simulink subsystem "PvtSubSys_LSM"  (R2020b)
settings: Solver=VariableStepAuto  StartTime=0.0  StopTime=10.0  RelTol=1e-3
values from neighbouring files (symbols this model uses):
  P_LSM_ALC_Enable = 0.0    [LSM_Parameter.sldd]
  P_LSM_DOP_C0_EN_Limit = 0.8    [LSM_Parameter.sldd]
  P_LSM_DOP_C0_out_Limit = 2.0    [LSM_Parameter.sldd]
  P_LSM_DOP_C1_EN_Limit : value not decoded    [LSM_Parameter.sldd]
  P_LSM_DOP_C1_out_Limit : value not decoded    [LSM_Parameter.sldd]
  P_LSM_DOP_C1AndC2_Lim_X : value not decoded    [LSM_Parameter.sldd]
  P_LSM_DOP_C2_EN_Limit : value not decoded    [LSM_Parameter.sldd]
  P_LSM_DOP_C2_out_Limit : value not decoded    [LSM_Parameter.sldd]
  P_LSM_DOP_In_Pre2Dop_Dis = 1.0    [LSM_Parameter.sldd]
  P_LSM_DOP_Out_Pre2Dop_Dis = 2.0    [LSM_Parameter.sldd]
  P_LSM_DOP_PreDis_X : value not decoded    [LSM_Parameter.sldd]
  P_LSM_DOP_PreDis_Y : value not decoded    [LSM_Parameter.sldd]
  P_LSM_DOPValid_CheckTime = 0.06    [LSM_Parameter.sldd]
  P_LSM_DoubleLine_Curr2Cent_Dislimit = 0.5    [LSM_Parameter.sldd]
  P_LSM_DoubleLine_Dop2Cent_Dislimit = 0.5    [LSM_Parameter.sldd]
  P_LSM_DoubleLine_DOPOut_C1 : value not decoded    [LSM_Parameter.sldd]
  P_LSM_DoubleLine_Pre2Cent_Dislimit = 1.0    [LSM_Parameter.sldd]
  P_LSM_IFV2CenterAxis = 0.0    [LSM_Parameter.sldd]
  P_LSM_IFV2RearAxis = 0.0    [LSM_Parameter.sldd]
  P_LSM_LineSTD_Limit = 0.15    [LSM_Parameter.sldd]
  P_LSM_NOH_Switch = 0.0    [LSM_Parameter.sldd]
  P_LSM_Pre_t = 0.0    [LSM_Parameter.sldd]
  P_LSM_SingleLine_Cent2Edge_Dislimit = 100.0    [LSM_Parameter.sldd]
  P_LSM_SingleLine_Curr2Cent_Dislimit = 0.2    [LSM_Parameter.sldd]
  P_LSM_SingleLine_Dop2Cent_Dislimit = 0.2    [LSM_Parameter.sldd]
  P_LSM_SingleLine_DOPOut_C1 : value not decoded    [LSM_Parameter.sldd]
  P_LSM_SingleLine_Pre2Cent_Dislimit = 0.5    [LSM_Parameter.sldd]
undefined symbols (not defined in the file or in its folder): P_LSM_LineWijCal_C12, P_LSM_LineWijCal_C13, P_LSM_PosLineLcFac
libraries: simulink x92, TrueDurationTime x2
(part 3 of 9)

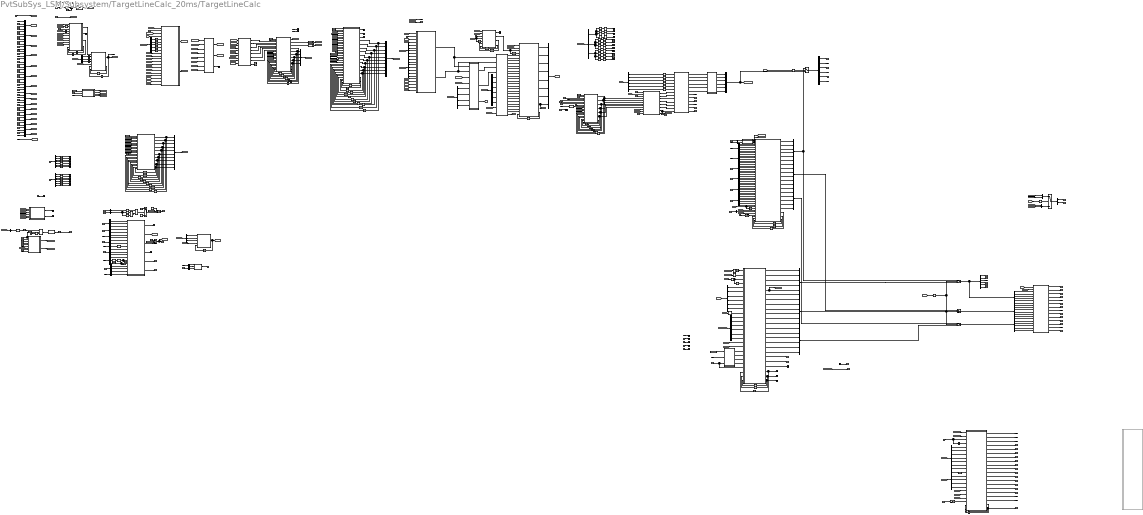
== system PvtSubSys_LSM/Subsystem/TargetLineCalc_20ms/TargetLineCalc ==
  kap : Inport
  vRef : Inport  Port=2
  OTLineValid : Inport  Port=3
  aOTL : Inport  Port=4
  bOTL : Inport  Port=5
  cOTL : Inport  Port=6
  dOTL : Inport  Port=7
  dxMax : Inport  Port=8
  OTLCount : Inport  Port=9
  ACCMode : Inport  Port=10
  HWASts : Inport  Port=11
  LRELineUpdate : Inport  Port=12
  LALineUpdate : Inport  Port=13
  LeftLine_Change : Inport  Port=14
  RightLine_Change : Inport  Port=15
  L1_Conf : Inport  Port=16
  L2_Conf : Inport  Port=17
  L3_Conf : Inport  Port=18
  L4_Conf : Inport  Port=19
  L1_A3 : Inport  Port=20
  L2_A3 : Inport  Port=21
  L3_A3 : Inport  Port=22
  L4_A3 : Inport  Port=23
  L1_A2 : Inport  Port=24
  L2_A2 : Inport  Port=25
  L3_A2 : Inport  Port=26
  L4_A2 : Inport  Port=27
  L1_A1 : Inport  Port=28
  L2_A1 : Inport  Port=29
  L3_A1 : Inport  Port=30
  L4_A1 : Inport  Port=31
  L1_A0 : Inport  Port=32
  L2_A0 : Inport  Port=33
  L3_A0 : Inport  Port=34
  L4_A0 : Inport  Port=35
  L1_R : Inport  Port=36
  L2_R : Inport  Port=37
  L3_R : Inport  Port=38
  L4_R : Inport  Port=39
  L1_Re : Inport  Port=40
  L2_Re : Inport  Port=41
  L3_Re : Inport  Port=42
  L4_Re : Inport  Port=43
  Edge1_R : Inport  Port=44
  Edge2_R : Inport  Port=45
  Edge1_A3 : Inport  Port=46
  Edge2_A3 : Inport  Port=47
  Edge1_A2 : Inport  Port=48
  Edge2_A2 : Inport  Port=49
  Edge1_A1 : Inport  Port=50
  Edge2_A1 : Inport  Port=51
  Edge1_A0 : Inport  Port=52
  Edge2_A0 : Inport  Port=53
  Edge1_Conf : Inport  Port=54
  Edge2_Conf : Inport  Port=55
  Edge1_Re : Inport  Port=56
  Edge2_Re : Inport  Port=57
  LeftLineType : Inport  Port=58
  RightLineType : Inport  Port=59
  LeftDLM : Inport  Port=60
  RightDLM : Inport  Port=61
  LH1Color : Inport  Port=62
  LH2Color : Inport  Port=63
  LeftDECELType : Inport  Port=64
  RightDECELType : Inport  Port=65
  LLeftType : Inport  Port=66
  pathPredValid : Inport  Port=67
  pathPredC3 : Inport  Port=68
  pathPredC2 : Inport  Port=69
  pathPredC1 : Inport  Port=70
  pathPredC0 : Inport  Port=71
  ESSSts : Inport  Port=72
  LCKSts : Inport  Port=73
  RFM_INTERSEC_ALERT : Inport  Port=74
  RFM_CURRENT_LANE : Inport  Port=75
  RFM_RIGHT_LANE : Inport  Port=76
  RFM_BRANCH : Inport  Port=77
  RFM_ROAD : Inport  Port=78  OutDataTypeStr=Bus: RFM_ROAD_BUS  PortDimensions=1  BusOutputAsStruct=on
  RFM_LINE_ENTRY_CL : Inport  Port=79
  RFM_LINE_EXIT_CL : Inport  Port=80
  RFM_LINE_CL : Inport  Port=81
  RFM_TSR_BUS : Inport  Port=82  OutDataTypeStr=Bus: RFM_TSR_BUS
  RFM_REC_LANES : Inport  Port=83
  RFM_LINE_L1 : Inport  Port=84
  RFM_LINE_R1 : Inport  Port=85
  RFM_LINE_L2 : Inport  Port=86
  RFM_LINE_R2 : Inport  Port=87
  Bus Creator : BusCreator  Inputs=10
  Bus Creator1 : BusCreator  Inputs=10
  Bus Creator10 : BusCreator  Inputs=2
  Bus Creator11 : BusCreator  Inputs=5
  Bus Creator12 : BusCreator  Inputs=8
  Bus Creator{2..8} (7 alike) : BusCreator  Inputs=6
  Bus Creator9 : BusCreator  Inputs=2
  Bus Selector : BusSelector  OutputSignals=LineConf,A1,A0
  Bus Selector1 : BusSelector  OutputSignals=LineConf
  Bus Selector{2,9..10,39} (4 alike) : BusSelector  OutputSignals=HWALineValid,HWALineC3,HWALineC2,HWALineC1,HWALineC0,HWARange
  Bus Selector11 : BusSelector  OutputSignals=b_is_avalible,en_lane_type
  Bus Selector12 : BusSelector  OutputSignals=b_is_available,f_distance,en_direction
  Bus Selector13 : BusSelector  OutputSignals=i_mapvalid
  Bus Selector14 : BusSelector  OutputSignals=nLaneNum,nLaneID
  Bus Selector15 : BusSelector  OutputSignals=b_vanish_valid
  Bus Selector{7,16,20..21,29} (5 alike) : BusSelector  OutputSignals=bIsLineExist,dC0V,dC1V,dC2V,dC3V,dDisFront
  Bus Selector17 : BusSelector  OutputSignals=dDisStart,bIsLineExist,dC0V
  Bus Selector18 : BusSelector  OutputSignals=bIsLineExist,dC0V,dC1V,dC2V,dC3V,dDisStart,dDisFront
  Bus Selector19 : BusSelector  OutputSignals=bIsLineExist,dC0V,dC1V,dC2V,dC3V,dDisStart,dDisFront
  Bus Selector22 : BusSelector  OutputSignals=Avail_time,Avail_dis,A0
  Bus Selector23 : BusSelector  OutputSignals=PathValid,PathA3,PathA2,PathA1,PathA0,PathRange
  Bus Selector24 : BusSelector  OutputSignals=RoadType
  Bus Selector25 : BusSelector  OutputSignals=HWALeLineValid,HWALeLineC3,HWALeLineC2,HWALeLineC1,HWALeLineC0,HWALeRange
  Bus Selector26 : BusSelector  OutputSignals=i_rec_lanes_num,i_rec_lanes
  Bus Selector27 : BusSelector  OutputSignals=eLineType
  Bus Selector28 : BusSelector  OutputSignals=eLineType
  Bus Selector3 : BusSelector  OutputSignals=LineConf,A3,A2,A1,A0,Range,tLost
  Bus Selector30 : BusSelector  OutputSignals=LineConf,A3,A2,A1,A0,LineReliable,Range
  Bus Selector31 : BusSelector  OutputSignals=RoadType,VehInLeftmostLane,VehInRightmostLane
  Bus Selector32 : BusSelector  OutputSignals=i_mapvalid,i_on_nav_path
  Bus Selector33 : BusSelector  OutputSignals=bIsLineExist,dDisStart,dC0V
  Bus Selector34 : BusSelector  OutputSignals=SPL_LaneChanged
  Bus Selector35 : BusSelector  OutputSignals=f_vanish_pt_dis
  Bus Selector36 : BusSelector  OutputSignals=HWARiLineValid,HWARiLineC3,HWARiLineC2,HWARiLineC1,HWARiLineC0,HWARiRange
  Bus Selector37 : BusSelector  OutputSignals=b_is_avalible
  Bus Selector38 : BusSelector  OutputSignals=LineValid,A3,A2,A1,A0
  Bus Selector4 : BusSelector  OutputSignals=EdgeConf,EdgeA3,EdgeA2,EdgeA1,EdgeA0
  Bus Selector40 : BusSelector  OutputSignals=LeftEn,RightEn
  Bus Selector41 : BusSelector  OutputSignals=LineValid,A3,A2,A1,A0
  Bus Selector42 : BusSelector  OutputSignals=LineConf,A3,A2,A1,A0,Range
  Bus Selector43 : BusSelector  OutputSignals=A3,A2,A1,A0
  Bus Selector5 : BusSelector  OutputSignals=EdgeConf,EdgeA1,EdgeA0
  Bus Selector6 : BusSelector  OutputSignals=PathValid,PathA3,PathA2,PathA1,PathA0,PathRange
  Bus Selector8 : BusSelector  OutputSignals=bIsLineExist,dC0V,dC1V,dC2V,dC3V,dDisFront,dDisStart
  CalcEgoVehMove : MATLAB Function  TreatAsAtomicUnit=on
  CalcEgoVehMove2 : MATLAB Function  TreatAsAtomicUnit=on
  Compare To Constant10 : simulink/Logic and Bit Operations/Compare To Constant  relop===  const=2  OutDataTypeStr=boolean
  Compare To Constant17 : simulink/Logic and Bit Operations/Compare To Constant  relop=~=  const=0  OutDataTypeStr=boolean
  Compare To Constant2 : simulink/Logic and Bit Operations/Compare To Constant  relop=~=  const=0  OutDataTypeStr=boolean
  Compare To Constant3 : simulink/Logic and Bit Operations/Compare To Constant  relop=~=  const=0  OutDataTypeStr=boolean
  Compare To Constant8 : simulink/Logic and Bit Operations/Compare To Constant  relop=>  const=0  OutDataTypeStr=boolean
  Compare To Constant9 : simulink/Logic and Bit Operations/Compare To Constant  relop===  const=1  OutDataTypeStr=boolean
  Compare To Zero : simulink/Logic and Bit Operations/Compare To Zero  relop=>  OutDataTypeStr=boolean
  Compare To Constant1 : simulink/Logic and Bit Operations/Compare To Constant  relop===  const=0  OutDataTypeStr=boolean
  Compare To Constant59 : simulink/Logic and Bit Operations/Compare To Constant  relop=~=  const=2  OutDataTypeStr=boolean
  Compare To Constant60 : simulink/Logic and Bit Operations/Compare To Constant  relop=>=  const=150  OutDataTypeStr=boolean
  Constant{,1..4} (5 alike) : Constant  Value=0.02  OutDataTypeStr=single
  Constant10 : Constant  Value=P_LSM_NOH_Switch
  Constant14 : Constant  Value=P_LSM_LineSTD_Limit
  Constant15 : Constant  Value=0  OutDataTypeStr=uint8
  Constant16 : Constant  Value=3  OutDataTypeStr=uint8
  Constant17 : Constant  Value=0  OutDataTypeStr=uint8
  Constant18 : Constant  Value=P_LSM_ALC_Enable  OutDataTypeStr=uint8
  Constant7 : Constant  Value=P_LSM_Pre_t
  Constant8 : Constant  Value=1.3  OutDataTypeStr=single
  Constant9 : Constant  Value=2  OutDataTypeStr=uint8
  D1 : Lookup_n-D  NumberOfTableDimensions=1  BreakpointsForDimension1=[0,30,40]  Table=[10,25,25]  InternalRulePriority=Speed  RndMeth=Simplest  InputSameDT=on
  D2 : Lookup_n-D  NumberOfTableDimensions=1  BreakpointsForDimension1=[0,30,40]  Table=[15,25,25]  InternalRulePriority=Speed  RndMeth=Simplest  InputSameDT=on
  Data Type Conversion{,1..3} (4 alike) : DataTypeConversion  OutDataTypeStr=boolean
  DetectChange : Subsystem
  DetectIncrease : Subsystem
  DetectIncrease1 : Subsystem
  ESSLineCalc : MATLAB Function  Commented=on  TreatAsAtomicUnit=on
  ESSLineCalc1 : MATLAB Function  TreatAsAtomicUnit=on
  Gain3 : Gain  Gain=3.6
  Gain4 : Gain  Gain=1.03
  Ground : Ground
  HWALineCalc : MATLAB Function  TreatAsAtomicUnit=on
  LCKSts1 : InportShadow  Port=73
  LH1Color1 : InportShadow  Port=62
  LREWidthCalc : MATLAB Function  TreatAsAtomicUnit=on
  LeftLineType1 : InportShadow  Port=58
  LineSelect : MATLAB Function  TreatAsAtomicUnit=on
  Logical Operator : Logic  Inputs=3  AllPortsSameDT=off  OutDataTypeStr=boolean
  Logical Operator7 : Logic  AllPortsSameDT=off  OutDataTypeStr=boolean
  Logical Operator8 : Logic  Operator=OR  AllPortsSameDT=off  OutDataTypeStr=boolean
  MATLAB Function : MATLAB Function  TreatAsAtomicUnit=on
  MATLAB Function1 : MATLAB Function  TreatAsAtomicUnit=on
  MATLAB Function2 : MATLAB Function  TreatAsAtomicUnit=on
  MATLAB Function3 : MATLAB Function  TreatAsAtomicUnit=on
  MATLAB Function4 : MATLAB Function  TreatAsAtomicUnit=on
  MATLAB Function5 : MATLAB Function  TreatAsAtomicUnit=on
  MATLAB Function6 : MATLAB Function  TreatAsAtomicUnit=on
  Mux{,1..6} (7 alike) : Mux
  Mux{7..15} (9 alike) : Mux  Inputs=2
  NOA : MATLAB Function  TreatAsAtomicUnit=on
  RFM_CURRENT_LANE1 : InportShadow  Port=75
  RFM_CURRENT_LANE2 : InportShadow  Port=75
  RFM_LINE_ENTRY_CL1 : InportShadow  Port=79
  RFM_LINE_EXIT_CL1 : InportShadow  Port=80
  RFM_LINE_EXIT_CL2 : InportShadow  Port=80
  RFM_LINE_L3 : InportShadow  Port=84
  RFM_LINE_R3 : InportShadow  Port=85
  RFM_ROAD1 : InportShadow  Port=78  OutDataTypeStr=Bus: RFM_ROAD_BUS  PortDimensions=1  BusOutputAsStruct=on
  RFM_ROAD2 : InportShadow  Port=78  OutDataTypeStr=Bus: RFM_ROAD_BUS  PortDimensions=1  BusOutputAsStruct=on
  RFM_TSR_BUS1 : InportShadow  Port=82  OutDataTypeStr=Bus: RFM_TSR_BUS
  RFM_TSR_BUS2 : InportShadow  Port=82  OutDataTypeStr=Bus: RFM_TSR_BUS
  RightLineType1 : InportShadow  Port=59
  RoadWidthCalc1 : MATLAB Function  TreatAsAtomicUnit=on
  Selector : Selector  InputPortWidth=4  IndexOptions=Index vector (dialog)  Indices=2  OutputSizes=1
  Selector{1,4..5,10} (4 alike) : Selector  InputPortWidth=4  IndexOptions=Index vector (dialog)  Indices=1  OutputSizes=1
  Selector11 : Selector  InputPortWidth=4  IndexOptions=Index vector (dialog)  Indices=4  OutputSizes=1
  Selector12 : Selector  InputPortWidth=4  IndexOptions=Index vector (dialog)  Indices=3  OutputSizes=1
  Selector{13..18} (6 alike) : Selector  InputPortWidth=3  IndexOptions=Index vector (dialog)  Indices=2  OutputSizes=1
  Selector2 : Selector  InputPortWidth=4  IndexOptions=Index vector (dialog)  Indices=3  OutputSizes=1
  Selector3 : Selector  InputPortWidth=4  IndexOptions=Index vector (dialog)  Indices=2  OutputSizes=1
  Selector6 : Selector  InputPortWidth=4  IndexOptions=Index vector (dialog)  Indices=4  OutputSizes=1
  Selector7 : Selector  InputPortWidth=4  IndexOptions=Index vector (dialog)  Indices=4  OutputSizes=1
  Selector8 : Selector  InputPortWidth=4  IndexOptions=Index vector (dialog)  Indices=3  OutputSizes=1
  Selector9 : Selector  InputPortWidth=4  IndexOptions=Index vector (dialog)  Indices=2  OutputSizes=1
  Signal Copy{,1..3,8,10..35} (31 alike) : SignalConversion  OverrideOpt=off
  Subsystem2 : Subsystem
  Subsystem3 : Subsystem
  Subsystem4 : Subsystem
  Subsystem5 : Subsystem
  Sum : Sum  Inputs=|++
  Switch{,1..6,9} (8 alike) : Switch  Criteria=u2 > Threshold
  TJA2NOA : MATLAB Function  TreatAsAtomicUnit=on
  Terminator{,1..49} (50 alike) : Terminator
  TrueDurationTime : TrueDurationTime/TrueDurationTime  TCycle=0.02
  TypeConf : Subsystem
  TypeConf1 : Subsystem
  Unit Delay{,1,6,10,13,15,27,30..32,34..35,39..41,49..52,58..59,64} (22 alike) : UnitDelay  SampleTime=-1  HasFrameUpgradeWarning=on
  Unit Delay11 : UnitDelay  InitialCondition=uint8(0)  SampleTime=-1  HasFrameUpgradeWarning=on
  Unit Delay12 : UnitDelay  InitialCondition=int8(0)  SampleTime=-1  HasFrameUpgradeWarning=on
  Unit Delay14 : UnitDelay  InitialCondition=3.75  SampleTime=-1  HasFrameUpgradeWarning=on
  Unit Delay16 : UnitDelay  InitialCondition=uint8(0)  SampleTime=-1  HasFrameUpgradeWarning=on
  Unit Delay{17..22,38} (7 alike) : UnitDelay  InitialCondition=single(zeros(2,1))  SampleTime=-1  HasFrameUpgradeWarning=on
  Unit Delay2 : UnitDelay  InitialCondition=[5;5;5;5]  SampleTime=-1  HasFrameUpgradeWarning=on
  Unit Delay23 : UnitDelay  InitialCondition=uint8(zeros(2,1))  SampleTime=-1  HasFrameUpgradeWarning=on
  Unit Delay24 : UnitDelay  InitialCondition=uint8(0)  SampleTime=-1  HasFrameUpgradeWarning=on
  Unit Delay25 : UnitDelay  InitialCondition=false  SampleTime=-1  HasFrameUpgradeWarning=on
  Unit Delay26 : UnitDelay  InitialCondition=int8(0)  SampleTime=-1  HasFrameUpgradeWarning=on
  Unit Delay{4..5,7..9,28..29,37,57,60..61} (11 alike) : UnitDelay  InitialCondition=zeros(4,1)  SampleTime=-1  HasFrameUpgradeWarning=on
  Unit Delay33 : UnitDelay  InitialCondition=3.75  SampleTime=-1  HasFrameUpgradeWarning=on
  Unit Delay36 : UnitDelay  InitialCondition=8  SampleTime=-1  HasFrameUpgradeWarning=on
  Unit Delay42 : UnitDelay  InitialCondition=false  SampleTime=-1  HasFrameUpgradeWarning=on
  Unit Delay{43..48,54,56,66..70} (13 alike) : UnitDelay  InitialCondition=single(0)  SampleTime=-1  HasFrameUpgradeWarning=on
  Unit Delay55 : UnitDelay  InitialCondition=false  SampleTime=-1  HasFrameUpgradeWarning=on
  Unit Delay62 : UnitDelay  InitialCondition=zeros(2,1)  SampleTime=-1  HasFrameUpgradeWarning=on
  Unit Delay63 : UnitDelay  InitialCondition=zeros(2,1)  SampleTime=-1  HasFrameUpgradeWarning=on
  Unit Delay65 : UnitDelay  InitialCondition=int8(0)  SampleTime=-1  HasFrameUpgradeWarning=on
  VehStation : MATLAB Function  TreatAsAtomicUnit=on
  VisLineFilter1 : MATLAB Function  TreatAsAtomicUnit=on
  VisLineFilter2 : MATLAB Function  TreatAsAtomicUnit=on
  VisLineFilter3 : MATLAB Function  TreatAsAtomicUnit=on
  VisLineFilter4 : MATLAB Function  TreatAsAtomicUnit=on
  VisLineFilter5 : MATLAB Function  TreatAsAtomicUnit=on
  YBranchRi : MATLAB Function  TreatAsAtomicUnit=on
  kap1 : InportShadow
  kap2 : InportShadow
  kap4 : InportShadow
  preDisMinTable : Lookup_n-D  NumberOfTableDimensions=1  BreakpointsForDimension1=[0 5 10 15 20 25 30 35 40 60 80 90 100 110 120 140]  Table=[8 9 10 11 12 13 14 15 17 22 28 31 35 38 42 49]  ExtrapMethod=Clip  InternalRulePriority=Speed  RndMeth=Simplest  InputSameDT=on
  tFilt : Constant  Value=0.2  OutDataTypeStr=single
  vRef{1..12,14} (13 alike) : InportShadow  Port=2
  TJALineValid : Outport
  TJALineA3 : Outport  Port=2
  TJALineA2 : Outport  Port=3
  TJALineA1 : Outport  Port=4
  TJALineA0 : Outport  Port=5
  TJALineRange : Outport  Port=6
  LCKLineValid : Outport  Port=7
  LCKLineA3 : Outport  Port=8
  LCKLineA2 : Outport  Port=9
  LCKLineA1 : Outport  Port=10
  LCKLineA0 : Outport  Port=11
  LCKLineRange : Outport  Port=12
  HWALineValid : Outport  Port=13
  HWALineA3 : Outport  Port=14
  HWALineA2 : Outport  Port=15
  HWALineA1 : Outport  Port=16
  HWALineA0 : Outport  Port=17
  HWALineRange : Outport  Port=18
  HWALineLValid1 : Outport  Port=19
  HWALineLA3 : Outport  Port=20
  HWALineLA2 : Outport  Port=21
  HWALineLA1 : Outport  Port=22
  HWALineLA0 : Outport  Port=23
  HWALineLRange : Outport  Port=24
  HWALineRValid : Outport  Port=25
  HWALineRA3 : Outport  Port=26
  HWALineRA2 : Outport  Port=27
  HWALineRA1 : Outport  Port=28
  HWALineRA0 : Outport  Port=29
  HWALineRRange0 : Outport  Port=30
  pre_dy_Error : Outport  Port=31
  pre_HeadAng_Error : Outport  Port=32
  MLeLane : Outport  Port=33
  RoadWidth : Outport  Port=34
  SingleLineLost_b : Outport  Port=35
  DoubleLineLost_b : Outport  Port=36
  LeLineCrossing : Outport  Port=37
  RiLineCrossing : Outport  Port=38
  MRiLane : Outport  Port=39
  MrcStopLane : Outport  Port=40
  HWALeLineVirtual : Outport  Port=41
  HWARiLineVirtual : Outport  Port=42
  LeLineLcAvailable : Outport  Port=43
  RiLineLcAvailable : Outport  Port=44
  ESSLineValid : Outport  Port=45
  ESSLineA3 : Outport  Port=46
  ESSLineA2 : Outport  Port=47
  ESSLineA1 : Outport  Port=48
  ESSLineA0 : Outport  Port=49
  ESSLineRange : Outport  Port=50
  ESSLineLValid : Outport  Port=51
  ESSLineLA3 : Outport  Port=52
  ESSLineLA2 : Outport  Port=53
  ESSLineLA1 : Outport  Port=54
  ESSLineLA0 : Outport  Port=55
  ESSLineLRange : Outport  Port=56
  ESSLineRValid : Outport  Port=57
  ESSLineRA3 : Outport  Port=58
  ESSLineRA2 : Outport  Port=59
  ESSLineRA1 : Outport  Port=60
  ESSLineRA0 : Outport  Port=61
  ESSLineRRange : Outport  Port=62
  ESSLineLock_b : Outport  Port=63
  leftLaneCurise_b : Outport  Port=64
  PilotSts : Outport  Port=65
  PilotTurnSwSts : Outport  Port=66
  PilotSPLDist : Outport  Port=67
  PilotSPL : Outport  Port=68
  TJALineSource : Outport  Port=69
  tag scope: RoadWidth=global, VisEdge=global, VisLine=global
  wires:
  [LH2Wij] -> VisLineFilter2/21(LH2Wij)
  [LH1Wij] -> VisLineFilter2/20(LH1Wij)
  Unit Delay35/1 -> RoadWidthCalc1/4(a0)
  Unit Delay59/1 -> RoadWidthCalc1/3(a1)
  Unit Delay58/1 -> RoadWidthCalc1/2(VisLineConf)
  Bus Selector/2 -> Unit Delay59/1  "<A1>"
  Bus Selector/1 -> Unit Delay58/1  "<LineConf>"
  Unit Delay13/1 -> YBranchRi/2(RightOffset_b)
  YBranchRi/2(YBranchRi_b) -> Terminator48/1
  Unit Delay12/1 -> VisLineFilter5/28(LockIDK1)
  VisLineFilter5/9(LockID) -> Unit Delay12/1
  MATLAB Function3/8(Line_State) -> Terminator41/1
  [RightOffset_b] -> VisLineFilter2/19(RightLineChange)
  [LeftOffset_b] -> VisLineFilter2/18(LeftLineChange)
  Ground/1 -> SingleLineLost_b/1  "SingleLineLost_b"
  kap1/1 -> Subsystem2/12(kap)
  Bus Selector37/1 -> MATLAB Function/3(Right_avail)  "<b_is_avalible>"
  RFM_RIGHT_LANE/1 -> Bus Selector37/1
  Bus Selector11/2 -> MATLAB Function/2(Cur_LaneType)  "<en_lane_type>"
  RFM_CURRENT_LANE2/1 -> Bus Selector11/1
  MATLAB Function/1(MrcStopLane) -> MrcStopLane/1
  Bus Selector11/1 -> MATLAB Function/1(Cur_avail)  "<b_is_avalible>"
  Subsystem2/7(TJA_Line_State) -> [TJA_Line_State], LineSelect/13(TJA_Line_State)  "LSM_TJA_Line_State"
  Subsystem2/6(OTL_Range) -> LineSelect/12(dxMax)
  Subsystem2/2(OTL_C3) -> LineSelect/8(aOTL)
  Subsystem2/1(OTL_Valid) -> LineSelect/7(OTLineValid)
  Subsystem2/4(OTL_C1) -> LineSelect/10(cOTL)
  Subsystem2/5(OTL_C0) -> LineSelect/11(dOTL)
  Subsystem2/3(OTL_C2) -> LineSelect/9(bOTL)
  [VisEdge] -> Subsystem2/11(EdgeLine)
  [CentLine] -> Subsystem2/10(CentLine)
  vRef2/1 -> Subsystem2/3(vRef)  "LSM_VRef"
  LCKSts1/1 -> Subsystem2/1(LCKSts)
  VisLineFilter1/3(A2) -> Unit Delay48/1, Subsystem2/6(DOP_C2)
  VisLineFilter1/5(A0) -> Subsystem2/8(DOP_C0), Unit Delay46/1
  VisLineFilter1/4(A1) -> Subsystem2/7(DOP_C1), Unit Delay47/1
  Unit Delay46/1 -> VisLineFilter1/18(A0K1)
  VisLineFilter1/7(tLost) -> Unit Delay44/1
  VisLineFilter1/6(Range) -> Subsystem2/9(DOP_Range), Unit Delay45/1
  Unit Delay44/1 -> VisLineFilter1/20(tLostK1)
  Unit Delay47/1 -> VisLineFilter1/17(A1K1)
  Unit Delay42/1 -> VisLineFilter1/14(LineValidK1)
  Unit Delay48/1 -> VisLineFilter1/16(A2K1)
  VisLineFilter1/1(LineValid) -> Subsystem2/4(DOP_Valid), Unit Delay42/1
  Unit Delay43/1 -> VisLineFilter1/15(A3K1)
  Unit Delay45/1 -> VisLineFilter1/19(RangeK1)
  VisLineFilter1/2(A3) -> Subsystem2/5(DOP_C3), Unit Delay43/1
  Constant2/1 -> VisLineFilter1/1(tCycle)
  aOTL/1 -> VisLineFilter1/4(aOTL)
  bOTL/1 -> VisLineFilter1/5(bOTL)
  cOTL/1 -> VisLineFilter1/6(cOTL)
  dxMax/1 -> VisLineFilter1/8(R)
  [dDeltaX] -> VisLineFilter1/10(dDeltaX)
  [dDeltaY] -> VisLineFilter1/11(dDeltaY)
  [CosOfPsi] -> VisLineFilter1/12(CosOfPsi)
  [SinOfPsi] -> VisLineFilter1/13(SinOfPsi)
  Unit Delay23/1 -> VisLineFilter4/15(EdgeConfK1)
  Unit Delay22/1 -> VisLineFilter4/17(EdgeA3K1)
  Unit Delay21/1 -> VisLineFilter4/18(EdgeA2K1)
  VisLineFilter4/1(EdgeConf) -> Unit Delay23/1, Bus Creator/1
  VisLineFilter4/3(EdgeA3) -> Unit Delay22/1, Bus Creator/3
  VisLineFilter4/4(EdgeA2) -> Bus Creator/4, Unit Delay21/1
  Unit Delay20/1 -> VisLineFilter4/19(EdgeA1K1)
  VisLineFilter4/5(EdgeA1) -> Bus Creator/5, Unit Delay20/1
  Unit Delay19/1 -> VisLineFilter4/20(EdgeA0K1)
  VisLineFilter4/6(EdgeA0) -> Bus Creator/6, Unit Delay19/1
  Unit Delay18/1 -> VisLineFilter4/21(EdgeRangeK1)
  VisLineFilter4/7(EdgeRange) -> Bus Creator/7, Unit Delay18/1
  Unit Delay17/1 -> VisLineFilter4/22(EdgetLostK1)
  [VisEdgeConf] -> VisLineFilter4/2(VisEdgeConf)
  Constant4/1 -> VisLineFilter4/1(tCycle)
  [VisEdgeA3] -> VisLineFilter4/4(a3)
  [VisEdgeA2] -> VisLineFilter4/5(a2)
  [VisEdgeA1] -> VisLineFilter4/6(a1)
  [VisEdgeA0] -> VisLineFilter4/7(a0)
  [VisEdgeRange] -> VisLineFilter4/8(R)
  [VisEdgeUpdate] -> VisLineFilter4/9(LineUpdate)
  [dDeltaX] -> VisLineFilter4/10(dDeltaX)
  [dDeltaY] -> VisLineFilter4/11(dDeltaY)
  [CosOfPsi] -> VisLineFilter4/12(CosOfPsi)
  [SinOfPsi] -> VisLineFilter4/13(SinOfPsi)
  vRef6/1 -> VisLineFilter4/14(vRef)  "LSM_VRef"
  LALineUpdate/1 -> [VisLineUpdate]
  LRELineUpdate/1 -> [VisEdgeUpdate]
  OTLineValid/1 -> VisLineFilter1/3(OTLineValid)
  OTLCount/1 -> DetectChange/1(OTLCount)
  DetectChange/1(Out1) -> VisLineFilter1/9(LineUpdate)
  Bus Creator/1 -> [VisEdge]
  ESSSts/1 -> ESSLineCalc1/3(ESSSts), Unit Delay24/1
  [VisLine] -> Bus Selector3/1
  Bus Selector3/3 -> ESSLineCalc1/7(A2)  "<A2>"
  Bus Selector3/2 -> ESSLineCalc1/6(A3)  "<A3>"
  Bus Selector3/1 -> ESSLineCalc1/5(LineConf)  "<LineConf>"
  [VisEdge] -> Bus Selector4/1
  Bus Selector4/2 -> ESSLineCalc1/13(EdgeA3)  "<EdgeA3>"
  Bus Selector4/1 -> Data Type Conversion1/1  "<EdgeConf>"
  Bus Selector4/3 -> ESSLineCalc1/14(EdgeA2)  "<EdgeA2>"
  [LeftOffset_b] -> ESSLineCalc1/17(LeftOffset_b)
  [RightOffset_b] -> ESSLineCalc1/18(RightOffset_b)
  [RoadWidth] -> ESSLineCalc1/19(RoadWidth)
  vRef3/1 -> D1/1  "LSM_VRef"
  D1/1 -> ESSLineCalc1/20(ESSDistLim)
  ESSLineCalc1/20(Lock_b) -> ESSLineLock_b/1, Unit Delay25/1
  Unit Delay25/1 -> ESSLineCalc1/22(Lock_bK1)
  ESSLineCalc1/19(MoveID) -> Unit Delay26/1
  Unit Delay26/1 -> ESSLineCalc1/21(MoveIDK1)
  ESSLineCalc1/17(ESSRiLineA0) -> ESSLineRA0/1
  ESSLineCalc1/16(ESSRiLineA1) -> ESSLineRA1/1
  ESSLineCalc1/15(ESSRiLineA2) -> ESSLineRA2/1
  ESSLineCalc1/14(ESSRiLineA3) -> ESSLineRA3/1
  ESSLineCalc1/11(ESSLeLineA0) -> ESSLineLA0/1
  ESSLineCalc1/1(ESSLineValid) -> ESSLineValid/1
  ESSLineCalc1/6(ESSRange) -> ESSLineRange/1
  ESSLineCalc1/7(ESSLeLineValid) -> ESSLineLValid/1
  ESSLineCalc1/2(ESSLineA3) -> ESSLineA3/1
  ESSLineCalc1/3(ESSLineA2) -> ESSLineA2/1
  ESSLineCalc1/4(ESSLineA1) -> ESSLineA1/1
  ESSLineCalc1/5(ESSLineA0) -> ESSLineA0/1
  ESSLineCalc1/8(ESSLeLineA3) -> ESSLineLA3/1
  ESSLineCalc1/9(ESSLeLineA2) -> ESSLineLA2/1
  ESSLineCalc1/10(ESSLeLineA1) -> ESSLineLA1/1
  ESSLineCalc1/12(ESSLeRange) -> ESSLineLRange/1
  ESSLineCalc1/13(ESSRiLineValid) -> ESSLineRValid/1
  ESSLineCalc1/18(ESSRiRange) -> ESSLineRRange/1
  Data Type Conversion1/1 -> ESSLineCalc1/12(EdgeValid)
  Unit Delay24/1 -> ESSLineCalc1/4(ESSStsK1)
  vRef/1 -> VisLineFilter2/15(vRef)  "LSM_VRef"
  [VisLineA3] -> VisLineFilter2/5(a3)
  VisLineFilter2/8(A1) -> Bus Creator1/5, Unit Delay7/1
  VisLineFilter2/6(A3) -> Bus Creator1/3, Unit Delay9/1
  VisLineFilter2/7(A2) -> Bus Creator1/4, Unit Delay8/1
  [CosOfPsi] -> VisLineFilter2/13(CosOfPsi)
  VisLineFilter2/11(tLost) -> Bus Creator1/8, Unit Delay2/1
  [SinOfPsi] -> VisLineFilter2/14(SinOfPsi)
  VisLineFilter2/3(DevDis) -> Terminator6/1
  [VisLineUpdate] -> VisLineFilter2/10(LineUpdate)
  Constant3/1 -> VisLineFilter2/2(tCycle)
  VisLineFilter2/2(DevAngle) -> Terminator5/1
  [VisLineA1] -> VisLineFilter2/7(a1)
  tFilt/1 -> VisLineFilter2/1(tF)
  VisLineFilter2/10(Range) -> Bus Creator1/7, Unit Delay4/1
  Unit Delay57/1 -> VisLineFilter2/22(LineConfK1)
  [dDeltaX] -> VisLineFilter2/11(dDeltaX)
  Unit Delay8/1 -> VisLineFilter2/25(A2K1)
  Unit Delay9/1 -> VisLineFilter2/24(A3K1)
  Unit Delay7/1 -> VisLineFilter2/26(A1K1)
  [VisLineR] -> VisLineFilter2/9(R)
  [VisLineConf] -> VisLineFilter2/3(VisLineConf)
  VisLineFilter2/1(DevValid) -> Terminator4/1
  Unit Delay5/1 -> VisLineFilter2/27(A0K1)
  VisLineFilter2/9(A0) -> Bus Creator1/6, Unit Delay5/1
  Bus Creator1/1 -> [VisLine]
  [VisLineA0] -> VisLineFilter2/8(a0)
  [RoadWidth] -> VisLineFilter2/17(RoadWidth)
  [dDeltaY] -> VisLineFilter2/12(dDeltaY)
  VisLineFilter2/4(LineConf) -> Bus Creator1/1, Unit Delay57/1
  Unit Delay2/1 -> VisLineFilter2/29(tLostK1)
  Unit Delay4/1 -> VisLineFilter2/28(RangeK1)
  [VisLineA2] -> VisLineFilter2/6(a2)
  YBranchRi/1(YBranch_b) -> RoadWidthCalc1/1(YBranch_b)
  [VisLineConf] -> YBranchRi/9(Conf)
  HWALineCalc/18(HWARiRange) -> Bus Creator7/6
  [VisLine] -> Bus Selector1/1
  Unit Delay34/1 -> YBranchRi/12(DistRiK1)
  Compare To Constant1/1 -> Logical Operator/1
  YBranchRi/4(DistRi) -> Unit Delay34/1
  Compare To Constant60/1 -> leftLaneCurise_b/1  "leftLaneCurise_b"
  Logical Operator/1 -> TrueDurationTime/1
  Compare To Constant59/1 -> Logical Operator/2
  [VisLineA2] -> YBranchRi/6(A2)
  TypeConf/1(Out1) -> [LeftLineTypeEN]  "LSM_LeftLineTypeEN"
  HWALineCalc/17(HWARiLineC0) -> Bus Creator7/5
  [RoadWidth] -> Unit Delay33/1
  HWALineCalc/19(preDyDiff) -> pre_dy_Error/1
  YBranchRi/3(Dist) -> Unit Delay32/1
  vRef12/1 -> YBranchRi/3(vRef)  "LSM_VRef"
  HWALineCalc/15(HWARiLineC2) -> Bus Creator7/3
  HWALineCalc/21(Error) -> Terminator/1
  RoadWidthCalc1/2(tLost) -> Unit Delay15/1
  RoadWidthCalc1/1(RoadWidth) -> RoadWidth/1, [RoadWidth], Unit Delay14/1
  [VisLineUpdate] -> RoadWidthCalc1/5(LineUpdate)
  [VisLineA1] -> YBranchRi/7(A1)
  [RightOffset_b] -> HWALineCalc/19(RightOffset_b)
  RightLineType/1 -> TypeConf/4(RightType)
  Unit Delay30/1 -> HWALineCalc/25(MoveIDK1)
  [LeftOffset_b] -> HWALineCalc/18(LeftOffset_b)
  HWALineCalc/16(HWARiLineC1) -> Bus Creator7/4
  CalcEgoVehMove2/2(dDeltaY) -> HWALineCalc/21(dDeltaY)
  Compare To Zero/1 -> Logical Operator/3
  Selector1/1 -> Compare To Constant1/1
  vRef7/1 -> HWALineCalc/24(vRef), CalcEgoVehMove2/3(Vego)  "LSM_VRef"
  HWALineCalc/20(HeadAngDiff) -> pre_HeadAng_Error/1
  Unit Delay16/1 -> HWALineCalc/4(HWAStsK1)
  vRef5/1 -> Compare To Zero/1  "LSM_VRef"
  Unit Delay15/1 -> RoadWidthCalc1/7(tLostK1)
  CalcEgoVehMove2/3(CosOfPsi) -> HWALineCalc/22(CosOfPsi)
  TrueDurationTime/1 -> Compare To Constant60/1
  Unit Delay33/1 -> YBranchRi/4(RoadWidth)
  Constant7/1 -> CalcEgoVehMove2/1(tCycle)
  [VisLineA3] -> YBranchRi/5(A3)
  kap4/1 -> CalcEgoVehMove2/2(Kap)
  CalcEgoVehMove2/4(SinOfPsi) -> HWALineCalc/23(SinOfPsi)
  [HWASts] -> Signal Copy/1
  Unit Delay14/1 -> RoadWidthCalc1/6(RoadWidthK1)
  HWALineCalc/14(HWARiLineC3) -> Bus Creator7/2
  TypeConf/2(Out2) -> [RightLineTypeEN]  "LSM_RightLineTypeEN"
  Bus Selector1/1 -> Selector1/1  "<LineConf>"
  [RightOffset_b] -> Unit Delay13/1
  HWALineCalc/13(HWARiLineValid) -> Bus Creator7/1
  [VisLine] -> Bus Selector/1
  LeftLineType/1 -> TypeConf/1(LeftType), Compare To Constant59/1
  [VisLineUpdate] -> YBranchRi/1(LineUpdate)
  HWALineCalc/22(MoveID) -> Terminator28/1, Unit Delay30/1  "LSM_MoveID"
  Unit Delay32/1 -> YBranchRi/11(DistK1)
  [VisLineA0] -> YBranchRi/8(A0)
  CalcEgoVehMove2/1(dDeltaX) -> HWALineCalc/20(dDeltaX)
  Constant/1 -> CalcEgoVehMove/1(tCycle)
  CalcEgoVehMove/1(dDeltaX) -> [dDeltaX]
  CalcEgoVehMove/3(CosOfPsi) -> [CosOfPsi]
  CalcEgoVehMove/4(SinOfPsi) -> [SinOfPsi]
  CalcEgoVehMove/2(dDeltaY) -> [dDeltaY]
  vRef1/1 -> CalcEgoVehMove/3(Vego)  "LSM_VRef"
  kap/1 -> CalcEgoVehMove/2(Kap)
  LeftDLM/1 -> TypeConf/2(LeftDLMType)
  RightDLM/1 -> TypeConf/5(RightDLMType)
  Bus Selector5/1 -> LREWidthCalc/1(LRELineConf)  "<EdgeConf>"
  Unit Delay36/1 -> LREWidthCalc/5(LREWidthK1)
  [VisEdge] -> Bus Selector5/1
  [VisEdgeUpdate] -> LREWidthCalc/4(LRELineUpdate)
  LREWidthCalc/1(LREWidth) -> [LREWidth], Unit Delay36/1
  [VisLineReliable] -> VisLineFilter2/4(VisLineReliable)
  VisLineFilter2/5(LineReliable) -> Bus Creator1/2, Unit Delay37/1
  Unit Delay37/1 -> VisLineFilter2/23(LineReliableK1)
  [VisEdgeReliable] -> VisLineFilter4/3(VisEdgeReliable)
  VisLineFilter4/2(EdgeReliable) -> Unit Delay38/1, Bus Creator/2
  Unit Delay38/1 -> VisLineFilter4/16(EdgeReliableK1)
  VisLineFilter4/8(EdgetLost) -> Unit Delay17/1, Bus Creator/8
  Bus Selector/3 -> Unit Delay35/1  "<A0>"
  Bus Selector5/2 -> LREWidthCalc/2(a1)  "<EdgeA1>"
  Bus Selector5/3 -> LREWidthCalc/3(a0)  "<EdgeA0>"
  Bus Selector3/4 -> ESSLineCalc1/8(A1)  "<A1>"
  Bus Selector3/5 -> ESSLineCalc1/9(A0)  "<A0>"
  Bus Selector3/6 -> ESSLineCalc1/10(Range)  "<Range>"
  Bus Selector3/7 -> ESSLineCalc1/11(tLost)  "<tLost>"
  Bus Selector4/4 -> ESSLineCalc1/15(EdgeA1)  "<EdgeA1>"
  Bus Selector4/5 -> ESSLineCalc1/16(EdgeA0)  "<EdgeA0>"
  Compare To Constant2/1 -> Switch3/2, Switch2/2, Switch/2
  HWALineCalc/3(HWALineC2) -> Bus Creator4/3
  HWALineCalc/6(HWARange) -> Bus Creator4/6
  Bus Creator3/1 -> Switch2/3
  Bus Selector10/1 -> HWALineValid/1  "<HWALineValid>"
  HWALineCalc/2(HWALineC3) -> Bus Creator4/2
  Bus Creator4/1 -> Switch/3
  HWALineCalc/9(HWALeLineC2) -> Bus Creator3/3
  Bus Selector10/2 -> HWALineA3/1  "<HWALineC3>"
  Bus Selector9/2 -> TJALineA3/1  "<HWALineC3>"
  HWALineCalc/12(HWALeRange) -> Bus Creator3/6
  HWALineCalc/5(HWALineC0) -> [HWALineC0], Bus Creator4/5
  Bus Selector10/6 -> HWALineRange/1  "<HWARange>"
  HWALineCalc/1(HWALineValid) -> Bus Creator4/1
  Bus Selector9/1 -> TJALineValid/1  "<HWALineValid>"
  Bus Selector10/3 -> HWALineA2/1  "<HWALineC2>"
  Bus Selector9/4 -> TJALineA1/1  "<HWALineC1>"
  Bus Selector9/3 -> TJALineA2/1  "<HWALineC2>"
  Bus Selector9/5 -> TJALineA0/1  "<HWALineC0>"
  Bus Creator2/1 -> Switch1/3, [TJA_Line]
  Switch1/1 -> Bus Selector9/1
  Bus Selector9/6 -> TJALineRange/1  "<HWARange>"
  HWALineCalc/8(HWALeLineC3) -> Bus Creator3/2
  HWALineCalc/10(HWALeLineC1) -> Bus Creator3/4
  HWALineCalc/11(HWALeLineC0) -> Bus Creator3/5
  HWALineCalc/7(HWALeLineValid) -> Bus Creator3/1
  Bus Selector10/5 -> HWALineA0/1  "<HWALineC0>"
  HWALineCalc/4(HWALineC1) -> Bus Creator4/4
  Bus Selector10/4 -> HWALineA1/1  "<HWALineC1>"
  TJA2NOA/1(HWALineValid) -> Bus Creator2/1
  TJA2NOA/2(HWALineC3) -> Bus Creator2/2
  TJA2NOA/3(HWALineC2) -> Bus Creator2/3
  TJA2NOA/4(HWALineC1) -> Bus Creator2/4
  TJA2NOA/5(HWALineC0) -> Bus Creator2/5
  TJA2NOA/6(HWARange) -> Bus Creator2/6
  VisLineFilter2/13(Avail_dis) -> Bus Creator1/10, Unit Delay60/1
  Unit Delay60/1 -> VisLineFilter2/31(Avail_disK1)
  VisLineFilter2/12(Avail_time) -> Bus Creator1/9, Unit Delay61/1
  Unit Delay61/1 -> VisLineFilter2/30(Avail_timeK1)
  Constant14/1 -> VisLineFilter2/16(Lowlimit)
  RFM_INTERSEC_ALERT/1 -> Bus Selector12/1
  RFM_ROAD/1 -> Bus Selector13/1
  Bus Selector12/1 -> Subsystem3/1(Intersec_available)  "<b_is_available>"
  Bus Selector12/2 -> Subsystem3/2(f_distance)  "<f_distance>"
  Bus Selector12/3 -> Subsystem3/3(en_direction)  "<en_direction>"
  Subsystem3/1(PilotRoadSts) -> Terminator42/1  "LSM_PilotTurnSwSts"
  Subsystem3/2(PilotTurnSwSts) -> [PilotRoadSts]  "LSM_PilotRoadSts"
  Subsystem3/3(PilotSts) -> Switch4/3  "LSM_PilotSts"
  [VisEdgeA0] -> VehStation/5(VisEdgeA0)
  [VisLineA0] -> VehStation/2(VisLineA0)
  [VisEdgeConf] -> VehStation/4(VisEdgeConf)
  [VisLineType] -> VehStation/3(VisLineType)
  [VisLineConf] -> VehStation/1(VisLineConf)
  Signal Copy8/1 -> Subsystem3/15(VehInLeftmostLane), MLeLane/1  "LSM_LeftMostLane"
  [PilotSts] -> Compare To Constant3/1
  RFM_LINE_ENTRY_CL/1 -> Bus Selector18/1
  RFM_LINE_EXIT_CL/1 -> Bus Selector17/1
  Subsystem3/6(PilotSPLDist) -> PilotSPLDist/1  "LSM_PilotSPLDist"
  Subsystem3/5(LSM_PilotSPL) -> PilotSPL/1  "LSM_PilotSPL"
  Bus Selector18/1 -> Signal Copy10/1  "<bIsLineExist>"
  Signal Copy10/1 -> Terminator1/1  "LSM_EN_Valid"
  Bus Selector18/4 -> Signal Copy13/1  "<dC2V>"
  Bus Selector18/3 -> Signal Copy12/1  "<dC1V>"
  Bus Selector18/2 -> Signal Copy11/1  "<dC0V>"
  Bus Selector18/5 -> Signal Copy14/1  "<dC3V>"
  Bus Selector18/6 -> Signal Copy15/1  "<dDisStart>"
  Bus Selector18/7 -> Signal Copy16/1  "<dDisFront>"
  Signal Copy11/1 -> Terminator7/1  "LSM_EN_C0"
  Signal Copy12/1 -> Terminator8/1  "LSM_EN_C1"
  Signal Copy13/1 -> Terminator9/1  "LSM_EN_C2"
  Signal Copy14/1 -> Terminator10/1  "LSM_EN_C3"
  Signal Copy15/1 -> Terminator11/1  "LSM_EN_Start"
  Signal Copy16/1 -> Terminator12/1  "LSM_EN_Front"
  Signal Copy23/1 -> Terminator16/1  "LSM_Exit_Front"
  Signal Copy22/1 -> Terminator15/1  "LSM_Exit_Start"
  Signal Copy21/1 -> Terminator14/1  "LSM_Exit_C3"
  Signal Copy20/1 -> Terminator19/1  "LSM_Exit_C2"
  Signal Copy19/1 -> Terminator18/1  "LSM_Exit_C1"
  Signal Copy18/1 -> Terminator17/1  "LSM_Exit_C0"
  Bus Selector19/7 -> Signal Copy23/1  "<dDisFront>"
  Bus Selector19/6 -> Signal Copy22/1  "<dDisStart>"
  Bus Selector19/5 -> Signal Copy21/1  "<dC3V>"
  Bus Selector19/2 -> Signal Copy18/1  "<dC0V>"
  Bus Selector19/3 -> Signal Copy19/1  "<dC1V>"
  Bus Selector19/4 -> Signal Copy20/1  "<dC2V>"
  Signal Copy17/1 -> Terminator13/1  "LSM_Exit_Valid"
  Bus Selector19/1 -> Signal Copy17/1  "<bIsLineExist>"
  RFM_LINE_EXIT_CL1/1 -> Bus Selector19/1
  VisLineFilter4/9(Avail_time) -> Bus Creator/9, Unit Delay63/1
  VisLineFilter4/10(Avail_dis) -> Bus Creator/10, Unit Delay62/1
  Unit Delay62/1 -> VisLineFilter4/24(Avail_disK1)
  Unit Delay63/1 -> VisLineFilter4/23(Avail_timeK1)
  HWALineCalc/24(Lock_counter) -> Terminator30/1, Unit Delay64/1  "LSM_LockCounter"
  Unit Delay64/1 -> HWALineCalc/27(Lock_counterK1)
  Unit Delay65/1 -> HWALineCalc/26(LockIDK1)
  HWALineCalc/23(LockID) -> Terminator29/1, Unit Delay65/1  "LSM_LockID"
  [VisLine] -> Bus Selector22/1
  Selector/1 -> Signal Copy25/1
  Selector2/1 -> Signal Copy24/1
  Bus Selector22/2 -> Selector4/1, Selector3/1, Selector7/1, Selector8/1  "<Avail_dis>"
  Selector4/1 -> Signal Copy26/1
  Selector3/1 -> Signal Copy27/1
  Signal Copy25/1 -> Terminator20/1  "LSM_L2_AvaliTime"
  Signal Copy24/1 -> Terminator21/1  "LSM_L3_AvaliTime"
  Signal Copy26/1 -> Terminator22/1  "LSM_L1_AvaliDis"
  Signal Copy27/1 -> Terminator23/1  "LSM_L2_AvaliDis"
  Signal Copy28/1 -> Terminator24/1  "LSM_L1_AvaliTime"
  Selector5/1 -> Signal Copy28/1
  Bus Selector22/1 -> Selector5/1, Selector/1, Selector2/1, Selector6/1  "<Avail_time>"
  Signal Copy29/1 -> Terminator25/1  "LSM_L4_AvaliTime"
  Selector6/1 -> Signal Copy29/1
  Signal Copy31/1 -> Terminator27/1  "LSM_L4_AvaliDis"
  Signal Copy30/1 -> Terminator26/1  "LSM_L3_AvaliDis"
  Selector7/1 -> Signal Copy31/1
  Selector8/1 -> Signal Copy30/1
  Selector12/1 -> Signal Copy34/1
  Selector11/1 -> Signal Copy35/1
  Signal Copy34/1 -> Terminator33/1  "LSM_L3_A0"
  Signal Copy35/1 -> Terminator34/1  "LSM_L4_A0"
  Signal Copy33/1 -> Terminator32/1  "LSM_L2_A0"
  Signal Copy32/1 -> Terminator31/1  "LSM_L1_A0"
  Selector9/1 -> Signal Copy33/1
  Selector10/1 -> Signal Copy32/1
  Bus Selector22/3 -> Selector12/1, Selector11/1, Selector9/1, Selector10/1  "<A0>"
  [LeftLineTypeEN] -> ESSLineCalc1/1(LeftLineTypeEn)
  [RightLineTypeEN] -> ESSLineCalc1/2(RightLineTypeEn)
  Unit Delay27/1 -> HWALineCalc/1(HWALineC0K1)  "LSM_HWALineC0K1"
  [VisLineReliable] -> YBranchRi/10(Reliable)
  VisLineFilter2/15(Fault) -> Unit Delay29/1
  VisLineFilter2/14(fix_time) -> Unit Delay28/1
  Unit Delay28/1 -> VisLineFilter2/32(fix_timeK1)
  Unit Delay29/1 -> VisLineFilter2/33(FaultK1)
  vRef11/1 -> Gain3/1  "LSM_VRef"
  Constant8/1 -> Sum/2
  Gain4/1 -> Sum/1
  Gain3/1 -> Gain4/1
  Sum/1 -> preDisMinTable/1
  preDisMinTable/1 -> [preDis]
  dOTL/1 -> VisLineFilter1/7(dOTL)
  vRef14/1 -> VisLineFilter1/2(vRef)  "LSM_VRef"
  [Line_State] -> Subsystem2/2(Line_State)
  kap2/1 -> [kap]
  LCKSts/1 -> MATLAB Function6/3(LCKSts)
  Switch4/1 -> [PilotSts], PilotSts/1
  Constant9/1 -> Switch4/1
  Constant10/1 -> Switch4/2
  [VisLineColor] -> VehStation/6(VisLineColor)
  VisLineFilter3/1(DoubleLineLost_b) -> [Double_Line_Lost]
  [Double_Line_Lost] -> DoubleLineLost_b/1  "DoubleLineLost_b"
  pathPredValid/1 -> Terminator36/1
  pathPredC3/1 -> Terminator37/1
  pathPredC2/1 -> Terminator38/1
  pathPredC1/1 -> Terminator39/1
  pathPredC0/1 -> Terminator40/1
  [CentLine] -> Bus Selector23/1
  Bus Selector23/3 -> HWALineCalc/7(PathA2)  "<PathA2>"
  Bus Selector23/2 -> HWALineCalc/6(PathA3)  "<PathA3>"
  Bus Selector23/4 -> HWALineCalc/8(PathA1)  "<PathA1>"
  Bus Selector23/1 -> HWALineCalc/5(PathValid)  "<PathValid>"
  Bus Selector23/5 -> HWALineCalc/9(PathA0)  "<PathA0>"
  Bus Selector23/6 -> HWALineCalc/10(PathRange)  "<PathRange>"
  Compare To Constant8/1 -> Logical Operator7/1
  Bus Selector24/1 -> Compare To Constant10/1, Compare To Constant9/1  "<RoadType>"
  Compare To Constant9/1 -> Logical Operator8/1
  Compare To Constant10/1 -> Logical Operator8/2
  Logical Operator7/1 -> Switch5/2
  Constant15/1 -> Switch5/1
  Switch5/1 -> Switch6/3
  Logical Operator8/1 -> Logical Operator7/2
  Constant16/1 -> Switch5/3
  Bus Selector13/1 -> Compare To Constant8/1  "<i_mapvalid>"
  RFM_TSR_BUS/1 -> Bus Selector24/1
  Switch6/1 -> PilotTurnSwSts/1
  Constant17/1 -> Switch6/1
  Constant18/1 -> Switch6/2
  RFM_REC_LANES/1 -> Bus Selector26/1
  Bus Selector26/1 -> Subsystem3/4(i_rec_lanes_num)  "<i_rec_lanes_num>"
  Bus Selector26/2 -> Subsystem3/5(i_rec_lanes)  "<i_rec_lanes>"
  RFM_ROAD1/1 -> Bus Selector14/1
  Bus Selector14/1 -> Subsystem3/6(nLaneNum)  "<nLaneNum>"
  Bus Selector14/2 -> Subsystem3/7(nLaneID)  "<nLaneID>"
  RFM_CURRENT_LANE/1 -> Bus Selector15/1
  Bus Selector15/1 -> Data Type Conversion/1  "<b_vanish_valid>"
  RFM_BRANCH/1 -> Terminator43/1
  Subsystem3/4(LaneChange) -> Terminator44/1
  Bus Selector8/7 -> NOA/33(Exit_Start)  "<dDisStart>"
  Bus Selector16/5 -> NOA/38(RFM_LineCL_A3)  "<dC3V>"
  Bus Selector21/6 -> NOA/26(RFM_LineR2_Range)  "<dDisFront>"
  Bus Selector7/3 -> NOA/11(RFM_LineL2_A1)  "<dC1V>"
  Bus Selector28/1 -> TypeConf1/2(RightType)  "<eLineType>"
  Unit Delay41/1 -> NOA/48(Lock_counterK1)
  RFM_LINE_CL/1 -> Bus Selector16/1
  RFM_LINE_R3/1 -> Bus Selector20/1
  NOA/21(Lock_counter) -> Unit Delay41/1
  Bus Selector20/1 -> NOA/15(RFM_LineR1_Valid)  "<bIsLineExist>"
  RFM_LINE_R1/1 -> Bus Selector28/1
  Bus Selector8/5 -> NOA/31(Exit_A3)  "<dC3V>"
  Bus Selector34/1 -> NOA/43(LaneChange)  "<SPL_LaneChanged>"
  NOA/4(HWALineC1) -> Bus Creator5/4
  RFM_LINE_L1/1 -> Bus Selector27/1
  NOA/5(HWALineC0) -> Bus Creator5/5
  Bus Selector20/4 -> NOA/18(RFM_LineR1_A2)  "<dC2V>"
  Bus Selector27/1 -> TypeConf1/1(LeftType)  "<eLineType>"
  RFM_LINE_L3/1 -> Bus Selector29/1
  Bus Selector8/1 -> NOA/27(Exit_Valid)  "<bIsLineExist>"
  Bus Selector8/4 -> NOA/30(Exit_A2)  "<dC2V>"
  NOA/17(HWARiLineC0) -> Bus Creator8/5
  Bus Selector16/2 -> NOA/35(RFM_LineCL_A0)  "<dC0V>"
  TypeConf1/2(RightEn) -> [RFM_RiLineLcAvailable], NOA/2(RightEn)
  Bus Selector21/5 -> NOA/25(RFM_LineR2_A3)  "<dC3V>"
  RFM_LINE_R2/1 -> Bus Selector21/1
  Bus Selector8/3 -> NOA/29(Exit_A1)  "<dC1V>"
  Bus Selector16/4 -> NOA/37(RFM_LineCL_A2)  "<dC2V>"
  Bus Selector8/2 -> NOA/28(Exit_A0)  "<dC0V>"
  NOA/15(HWARiLineC2) -> Bus Creator8/3
  Bus Selector20/6 -> NOA/20(RFM_LineR1_Range)  "<dDisFront>"
  Bus Selector7/6 -> NOA/14(RFM_LineL2_Range)  "<dDisFront>"
  Bus Selector21/4 -> NOA/24(RFM_LineR2_A2)  "<dC2V>"
  Bus Selector21/1 -> NOA/21(RFM_LineR2_Valid)  "<bIsLineExist>"
  Bus Selector8/6 -> NOA/32(Exit_Range)  "<dDisFront>"
  Bus Selector20/3 -> NOA/17(RFM_LineR1_A1)  "<dC1V>"
  RFM_LINE_EXIT_CL2/1 -> Bus Selector8/1
  Bus Selector16/1 -> NOA/34(RFM_LineCL_Valid)  "<bIsLineExist>"
  Bus Selector29/2 -> NOA/4(RFM_LineL1_A0)  "<dC0V>"
  RFM_LINE_L2/1 -> Bus Selector7/1
  [HWASts] -> Unit Delay39/1, NOA/40(HWASts)
  NOA/7(HWALeLineValid) -> Bus Creator6/1
  Bus Selector29/1 -> NOA/3(RFM_LineL1_Valid)  "<bIsLineExist>"
  Bus Selector21/3 -> NOA/23(RFM_LineR2_A1)  "<dC1V>"
  Unit Delay39/1 -> NOA/41(HWAStsK1)
  Bus Selector29/6 -> NOA/8(RFM_LineL1_Range)  "<dDisFront>"
  Bus Selector16/6 -> NOA/39(RFM_LineCL_Range)  "<dDisFront>"
  NOA/16(HWARiLineC1) -> Bus Creator8/4
  NOA/19(MoveID) -> Unit Delay40/1
  Bus Selector20/2 -> NOA/16(RFM_LineR1_A0)  "<dC0V>"
  NOA/20(LockID) -> Unit Delay/1
  NOA/14(HWARiLineC3) -> Bus Creator8/2
  Unit Delay40/1 -> NOA/46(MoveIDK1)
  D2/1 -> NOA/45(DistanceLim)
  NOA/11(HWALeLineC0) -> Bus Creator6/5
  Bus Selector16/3 -> NOA/36(RFM_LineCL_A1)  "<dC1V>"
  [PilotSts] -> NOA/42(PilotSts)
  TypeConf1/1(LeftEn) -> [RFM_LeLineLcAvailable], NOA/1(LeftEn)
  Bus Selector29/3 -> NOA/5(RFM_LineL1_A1)  "<dC1V>"
  Unit Delay/1 -> NOA/47(LockIDK1)
  NOA/8(HWALeLineC3) -> Bus Creator6/2
  Bus Selector7/5 -> NOA/13(RFM_LineL2_A3)  "<dC3V>"
  NOA/1(HWALineValid) -> Bus Creator5/1
  NOA/3(HWALineC2) -> Bus Creator5/3
  Bus Selector20/5 -> NOA/19(RFM_LineR1_A3)  "<dC3V>"
  Bus Selector7/1 -> NOA/9(RFM_LineL2_Valid)  "<bIsLineExist>"
  vRef8/1 -> D2/1  "LSM_VRef"
  Bus Selector7/2 -> NOA/10(RFM_LineL2_A0)  "<dC0V>"
  NOA/12(HWALeRange) -> Bus Creator6/6
  Bus Selector21/2 -> NOA/22(RFM_LineR2_A0)  "<dC0V>"
  [PilotRoadSts] -> NOA/44(PilotRoadSts)
  NOA/18(HWARiRange) -> Bus Creator8/6
  NOA/2(HWALineC3) -> Bus Creator5/2
  NOA/10(HWALeLineC1) -> Bus Creator6/4
  NOA/6(HWARange) -> Bus Creator5/6
  NOA/13(HWARiLineValid) -> Bus Creator8/1
  Bus Selector29/4 -> NOA/6(RFM_LineL1_A2)  "<dC2V>"
  Bus Selector29/5 -> NOA/7(RFM_LineL1_A3)  "<dC3V>"
  Bus Selector7/4 -> NOA/12(RFM_LineL2_A2)  "<dC2V>"
  NOA/9(HWALeLineC2) -> Bus Creator6/3
  Bus Creator5/1 -> Switch1/1, Switch/1
  Bus Creator6/1 -> Switch2/1
  [PilotSts] -> Compare To Constant2/1
  Bus Creator7/1 -> Switch3/3
  Bus Creator8/1 -> Switch3/1
  Compare To Constant3/1 -> Switch1/2
  RFM_TSR_BUS1/1 -> Bus Selector31/1
  RFM_ROAD2/1 -> Bus Selector32/1
  Bus Selector32/1 -> Subsystem3/8(i_mapvalid)  "<i_mapvalid>"
  Bus Selector32/2 -> Subsystem3/9(i_on_nav_path)  "<i_on_nav_path>"
  Bus Selector17/1 -> Subsystem3/11(" Exit_dDisStart")  "<dDisStart>"
  Bus Selector17/2 -> Subsystem3/12(ExitLineExist)  "<bIsLineExist>"
  Bus Selector17/3 -> Subsystem3/13(" Exit_dC0V")  "<dC0V>"
  Bus Selector31/1 -> Subsystem3/14(RoadType)  "<RoadType>"
  Bus Selector31/3 -> Data Type Conversion3/1  "<VehInRightmostLane>"
  RFM_LINE_ENTRY_CL1/1 -> Bus Selector33/1
  Bus Selector33/1 -> Subsystem3/17(Entry_bIsLineExist)  "<bIsLineExist>"
  Bus Selector33/2 -> Subsystem3/18(Entry_dDisStart)  "<dDisStart>"
  Bus Selector33/3 -> Subsystem3/19(Entry_dC0V)  "<dC0V>"
  Bus Selector31/2 -> Data Type Conversion2/1  "<VehInLeftmostLane>"
  VehStation/1(LeftMostLane) -> Terminator45/1
  VehStation/2(RightMostLane) -> Terminator46/1
  RFM_TSR_BUS2/1 -> Bus Selector34/1
  Data Type Conversion3/1 -> Subsystem3/16(VehInRightmostLane), MRiLane/1
  Data Type Conversion/1 -> Subsystem3/10(" b_vanish_valid")
  Data Type Conversion2/1 -> Signal Copy8/1
  Bus Selector35/1 -> Subsystem3/20(" f_vanish_pt_dis ")  "<f_vanish_pt_dis>"
  RFM_CURRENT_LANE1/1 -> Bus Selector35/1
  [VisLineUpdate] -> TypeConf/7(Line_update)
  Bus Selector6/1 -> Selector13/1  "<PathValid>"
  Bus Selector6/2 -> Selector14/1  "<PathA3>"
  Bus Selector6/3 -> Selector15/1  "<PathA2>"
  Bus Selector6/4 -> Selector16/1  "<PathA1>"
  Bus Selector6/5 -> Selector17/1  "<PathA0>"
  Bus Selector6/6 -> Selector18/1  "<PathRange>"
  LineSelect/1(TJALineValid) -> TJA2NOA/1(TJALineValid)
  LineSelect/2(TJALineA3) -> TJA2NOA/2(TJALineA3)
  LineSelect/3(TJALineA2) -> TJA2NOA/3(TJALineA2)
  LineSelect/4(TJALineA1) -> TJA2NOA/4(TJALineA1)
  LineSelect/5(TJALineA0) -> TJA2NOA/5(TJALineA0)
  LineSelect/6(TJALineRange) -> TJA2NOA/6(TJALineRange)
  LineSelect/7(LCKLineValid) -> LCKLineValid/1
  LineSelect/8(LCKLineA3) -> LCKLineA3/1
  LineSelect/9(LCKLineA2) -> LCKLineA2/1
  LineSelect/10(LCKLineA1) -> LCKLineA1/1
  LineSelect/11(LCKLineA0) -> LCKLineA0/1
  LineSelect/12(LCKLineRange) -> LCKLineRange/1
  ACCMode/1 -> Terminator47/1
  Subsystem2/8(Line_source) -> TJALineSource/1  "LSM_Line_source"
  LeftDECELType/1 -> TypeConf/3(LeftDECELType)
  RightDECELType/1 -> TypeConf/6(RightDECELType)
  Bus Selector25/5 -> MATLAB Function1/13(LeLineC0)  "<HWALeLineC0>"
  Switch3/1 -> Bus Selector36/1
  Bus Selector36/6 -> MATLAB Function1/20(RiLineRange)  "<HWARiRange>"
  MATLAB Function1/13(HWARiLineRange) -> HWALineRRange0/1
  Bus Selector39/6 -> MATLAB Function1/8(LineRange)  "<HWARange>"
  Switch2/1 -> Bus Selector25/1
  MATLAB Function1/14(RiLineVirtual_b) -> HWARiLineVirtual/1
  Bus Selector36/3 -> MATLAB Function1/17(RiLineC2)  "<HWARiLineC2>"
  Bus Selector25/2 -> MATLAB Function1/10(LeLineC3)  "<HWALeLineC3>"
  Bus Selector39/3 -> MATLAB Function1/5(LineC2)  "<HWALineC2>"
  MATLAB Function1/2(HWALeLineC3) -> HWALineLA3/1
  Bus Selector39/4 -> MATLAB Function1/6(LineC1)  "<HWALineC1>"
  [RoadWidth] -> MATLAB Function1/2(RoadWidth)
  MATLAB Function1/7(LeLineVirtual_b) -> HWALeLineVirtual/1
  MATLAB Function1/1(HWALeLineValid) -> HWALineLValid1/1
  MATLAB Function1/5(HWALeLineC0) -> HWALineLA0/1
  MATLAB Function1/4(HWALeLineC1) -> HWALineLA1/1
  MATLAB Function1/9(HWARiLineC3) -> HWALineRA3/1
  Bus Selector39/2 -> MATLAB Function1/4(LineC3)  "<HWALineC3>"
  Bus Selector25/6 -> MATLAB Function1/14(LeLineRange)  "<HWALeRange>"
  Bus Selector25/3 -> MATLAB Function1/11(LeLineC2)  "<HWALeLineC2>"
  Bus Selector25/1 -> MATLAB Function1/9(LeLineValid)  "<HWALeLineValid>"
  MATLAB Function1/10(HWARiLineC2) -> HWALineRA2/1
  Bus Selector36/5 -> MATLAB Function1/19(RiLineC0)  "<HWARiLineC0>"
  MATLAB Function1/11(HWARiLineC1) -> HWALineRA1/1
  [HWASts] -> MATLAB Function1/1(HWASts)
  Bus Selector36/2 -> MATLAB Function1/16(RiLineC3)  "<HWARiLineC3>"
  Switch/1 -> Bus Selector10/1, Bus Selector39/1
  Bus Selector36/4 -> MATLAB Function1/18(RiLineC1)  "<HWARiLineC1>"
  MATLAB Function1/12(HWARiLineC0) -> HWALineRA0/1
  MATLAB Function1/8(HWARiLineValid) -> HWALineRValid/1
  Bus Selector36/1 -> MATLAB Function1/15(RiLineValid)  "<HWARiLineValid>"
  Bus Selector25/4 -> MATLAB Function1/12(LeLineC1)  "<HWALeLineC1>"
  Bus Selector39/1 -> MATLAB Function1/3(LineValid)  "<HWALineValid>"
  Bus Selector39/5 -> MATLAB Function1/7(LineC0)  "<HWALineC0>"
  MATLAB Function1/6(HWALeLineRange) -> HWALineLRange/1
  MATLAB Function1/3(HWALeLineC2) -> HWALineLA2/1
  HWASts/1 -> [HWASts]
  [LeftLineTypeEN] -> Bus Creator10/1  "LeftEn"
  Bus Selector40/1 -> LeLineLcAvailable/1  "<LeftEn>"
  Compare To Constant17/1 -> Switch9/2
  Bus Creator9/1 -> Switch9/1
  Bus Selector40/2 -> RiLineLcAvailable/1  "<RightEn>"
  Switch9/1 -> Bus Selector40/1
  Bus Creator10/1 -> Switch9/3
  [RFM_LeLineLcAvailable] -> Bus Creator9/1  "LeftEn"
  [RFM_RiLineLcAvailable] -> Bus Creator9/2  "RightEn"
  [PilotSts] -> Compare To Constant17/1
  [RightLineTypeEN] -> Bus Creator10/2  "RightEn"
  LH1Color1/1 -> TypeConf/8(LeftColor)
  LLeftType/1 -> TypeConf/9(LLeftType)
  [CosOfPsi] -> Subsystem5/17(CosOfPsi)
  [SinOfPsi] -> Subsystem5/18(SinOfPsi)
  [dDeltaX] -> Subsystem5/19(dDeltaX)
  [dDeltaY] -> Subsystem5/20(dDeltaY)
  Mux/1 -> [VisLineConf]
  Mux1/1 -> [VisLineA3]
  Mux2/1 -> [VisLineA2]
  Mux3/1 -> [VisLineA1]
  Mux4/1 -> [VisLineA0]
  Mux5/1 -> [VisLineR]
  Mux6/1 -> [VisLineReliable]
  Mux7/1 -> [VisLineType]
  Mux8/1 -> [VisLineColor]
  [VisLineConf] -> Subsystem5/10(Conf)
  [VisLineA3] -> Subsystem5/11(<A3>)
  [VisLineA2] -> Subsystem5/12(<A2>)
  [VisLineA1] -> Subsystem5/13(<A1>)
  [VisLineA0] -> Subsystem5/14(<A0>)
  [VisLineReliable] -> Subsystem5/15(<LineReliable>)
  [VisLineR] -> Subsystem5/16(<Range>)
  Unit Delay31/1 -> Subsystem5/6(<CentLineC3>)
  Unit Delay49/1 -> Subsystem5/7(<CentLineC2>)
  Unit Delay50/1 -> Subsystem5/8(<CentLineC1>)
  Unit Delay51/1 -> Subsystem5/9(<CentLineC0>)
  Unit Delay52/1 -> Subsystem5/5(<CentLineValid>)
  [RoadWidth] -> Subsystem5/4(RoadWidth1)
  [LH1Wij] -> MATLAB Function2/1(LH1Wij)
  [LH2Wij] -> MATLAB Function2/2(LH2Wij)
  MATLAB Function2/1(LH1_Valid) -> [LH1Valid]
  MATLAB Function2/2(LH2_Valid) -> [LH2Valid]
  [LH1Valid] -> MATLAB Function3/1(LH1_Valid)
  [LH2Valid] -> MATLAB Function3/2(LH2_Valid)
  [CosOfPsi] -> VisLineFilter3/14(CosOfPsi)  "LSM_CosOfPsi"
  Unit Delay68/1 -> VisLineFilter3/21(A0K1)  "LSM_A0K1"
  Unit Delay69/1 -> VisLineFilter3/20(A1K1)  "LSM_A1K1"
  Unit Delay66/1 -> VisLineFilter3/23(tLostK1)  "LSM_tLostK1"
  [SinOfPsi] -> VisLineFilter3/15(SinOfPsi)  "LSM_SinOfsi"
  Unit Delay70/1 -> VisLineFilter3/19(A2K1)  "LSM_A2K1"
  VisLineFilter3/9(A0) -> Unit Delay68/1, Bus Creator11/5
  VisLineFilter3/10(Range) -> Unit Delay67/1
  [dDeltaY] -> VisLineFilter3/13(dDeltaY)  "LSM_dDeltaY"
  [dDeltaX] -> VisLineFilter3/12(dDeltaX)  "LSM_dDeltaX"
  Unit Delay67/1 -> VisLineFilter3/22(RangeK1)  "LSM_RangeK1"
  VisLineFilter3/11(tLost) -> Unit Delay66/1
  VisLineFilter3/6(A3) -> Unit Delay56/1, Bus Creator11/2
  Unit Delay54/1 -> VisLineFilter3/16(QualityK1)  "LSM_QualityK1"
  Unit Delay55/1 -> VisLineFilter3/17(LineValidK1)  "LSM_LineValidK1"
  VisLineFilter3/8(A1) -> Unit Delay69/1, Bus Creator11/4
  Unit Delay56/1 -> VisLineFilter3/18(A3K1)  "LSM_A3K1"
  VisLineFilter3/5(LineValid) -> Unit Delay55/1, Bus Creator11/1
  VisLineFilter3/4(Quality) -> Unit Delay54/1
  VisLineFilter3/7(A2) -> Bus Creator11/3, Unit Delay70/1
  Constant1/1 -> VisLineFilter3/1(tCycle)
  MATLAB Function3/1(CentLineValid) -> VisLineFilter3/3(CentLineValid)  "LSM_CentLineValid"
  MATLAB Function3/2(CentLineC3) -> VisLineFilter3/4(CentLineA3)  "LSM_CentLineA3"
  MATLAB Function3/3(CentLineC2) -> VisLineFilter3/5(CentLineA2)  "LSM_CentLineA2"
  MATLAB Function3/4(CentLineC1) -> VisLineFilter3/6(CentLineA1)  "LSM_CentLineA1"
  MATLAB Function3/5(CentLineC0) -> VisLineFilter3/7(CentLineA0)  "LSM_CentLineA0"
  MATLAB Function3/6(CentLineRange) -> VisLineFilter3/8(CentLineRange)  "LSM_CentLineRange"
  MATLAB Function3/7(CentLineReliable) -> VisLineFilter3/9(CentQ)  "LSM_CentQ"
  [VisLineUpdate] -> VisLineFilter3/11(LineUpdate)  "LSM_VisLineUpdate"
  [LeftOffset_b] -> LeLineCrossing/1
  [RightOffset_b] -> RiLineCrossing/1
  [VisLineA3] -> MATLAB Function3/3(VisLineA3)
  [VisLineA2] -> MATLAB Function3/4(VisLineA2)
  [VisLineA1] -> MATLAB Function3/5(VisLineA1)
  [VisLineA0] -> MATLAB Function3/6(VisLineA0)
  [VisLineR] -> MATLAB Function3/7(VisLineR)
  [VisLineA0] -> MATLAB Function2/8(VisLineA0)
  [VisLineA1] -> MATLAB Function2/7(VisLineA1)
  [VisLineA2] -> MATLAB Function2/6(VisLineA2)
  [VisLineA3] -> MATLAB Function2/5(VisLineA3)
  [preDis] -> Subsystem5/3(preDis)
  [preDis] -> MATLAB Function2/4(preDis)
  [preDis] -> Subsystem4/3(preDis)
  [RoadWidth] -> Subsystem4/4(RoadWidth1)
  Bus Selector41/1 -> Subsystem4/5(<CentLineValid>)  "<LineValid>"
  Bus Selector41/5 -> Subsystem4/9(<CentLineC0>)  "<A0>"
  Bus Selector41/4 -> Subsystem4/8(<CentLineC1>)  "<A1>"
  Bus Selector41/3 -> Subsystem4/7(<CentLineC2>)  "<A2>"
  Bus Selector41/2 -> Subsystem4/6(<CentLineC3>)  "<A3>"
  Bus Selector30/7 -> Subsystem4/16(<Range>)  "<Range>"
  Bus Selector30/6 -> Subsystem4/15(<LineReliable>)  "<LineReliable>"
  Bus Selector30/5 -> Subsystem4/14(<A0>)  "<A0>"
  Bus Selector30/4 -> Subsystem4/13(<A1>)  "<A1>"
  Bus Selector30/3 -> Subsystem4/12(<A2>)  "<A2>"
  Bus Selector30/2 -> Subsystem4/11(<A3>)  "<A3>"
  Bus Selector30/1 -> Subsystem4/10(Conf)  "<LineConf>"
  [dDeltaY] -> Subsystem4/20(dDeltaY)
  [dDeltaX] -> Subsystem4/19(dDeltaX)
  [SinOfPsi] -> Subsystem4/18(SinOfPsi)
  [CosOfPsi] -> Subsystem4/17(CosOfPsi)
  [VisLine] -> Bus Selector30/1
  Bus Creator11/1 -> [CentLineRef]
  [CentLineRef] -> Bus Selector38/1
  Bus Selector38/1 -> Unit Delay52/1  "<LineValid>"
  Bus Selector38/2 -> Unit Delay31/1  "<A3>"
  Bus Selector38/3 -> Unit Delay49/1  "<A2>"
  Bus Selector38/4 -> Unit Delay50/1  "<A1>"
  Bus Selector38/5 -> Unit Delay51/1  "<A0>"
  [CentLineRef] -> Bus Selector41/1
  Subsystem5/1(LH1Wij) -> [LH1Wij]
  Subsystem5/2(LH2Wij) -> [LH2Wij]
  [preDis] -> MATLAB Function5/4(preDis)
  Bus Selector43/1 -> MATLAB Function5/5(VisLineA3)  "<A3>"
  Bus Selector43/2 -> MATLAB Function5/6(VisLineA2)  "<A2>"
  Bus Selector43/3 -> MATLAB Function5/7(VisLineA1)  "<A1>"
  Bus Selector43/4 -> MATLAB Function5/8(VisLineA0)  "<A0>"
  MATLAB Function5/2(LH2_Valid) -> MATLAB Function4/4(LH2_Valid)  "LSM_LH2Valid"
  MATLAB Function5/1(LH1_Valid) -> MATLAB Function4/3(LH1_Valid)  "LSM_LH1Valid"
  Subsystem4/2(LH2Wij) -> MATLAB Function5/2(LH2Wij), MATLAB Function4/2(LH2Wij)  "LSM_LH2Wij"
  Subsystem4/1(LH1Wij) -> MATLAB Function5/1(LH1Wij), MATLAB Function4/1(LH1Wij)  "LSM_LH1Wij"
  [VisLine] -> Bus Selector42/1
  [VisLine] -> Bus Selector43/1
  Bus Selector42/2 -> MATLAB Function4/6(VisLineA3)  "<A3>"
  Bus Selector42/3 -> MATLAB Function4/7(VisLineA2)  "<A2>"
  Bus Selector42/4 -> MATLAB Function4/8(VisLineA1)  "<A1>"
  Bus Selector42/5 -> MATLAB Function4/9(VisLineA0)  "<A0>"
  Bus Selector42/6 -> MATLAB Function4/10(VisLineR)  "<Range>"
  [RightOffset_b] -> MATLAB Function6/2(RightOffset_b)
  [LeftOffset_b] -> MATLAB Function6/1(LeftOffset_b)
  MATLAB Function6/4(Cnt2) -> Unit Delay1/1
  Unit Delay1/1 -> MATLAB Function6/7(Cnt2K1)
  Unit Delay6/1 -> MATLAB Function6/6(Cnt1K1)
  MATLAB Function6/3(Cnt1) -> Unit Delay6/1
  MATLAB Function6/1(LaneChangeCancel_b) -> Terminator35/1
  MATLAB Function6/2(LckLock_b) -> VisLineFilter5/3(LckLock_b), Unit Delay10/1
  Bus Selector42/1 -> MATLAB Function4/5(VisLineConf)  "<LineConf>"
  [LeftOffset_b] -> VisLineFilter5/1(LeftOffset_b)
  [RightOffset_b] -> VisLineFilter5/2(RightOffset_b)
  Unit Delay10/1 -> VisLineFilter5/4(LckLock_bK1)
  MATLAB Function4/3(CentLineC2) -> VisLineFilter5/7(CentLineC2)
  MATLAB Function4/2(CentLineC3) -> VisLineFilter5/6(CentLineC3)
  MATLAB Function4/4(CentLineC1) -> VisLineFilter5/8(CentLineC1)
  MATLAB Function4/8(LeftLineValid) -> VisLineFilter5/12(LeftLineValid)
  MATLAB Function4/1(CentLineValid) -> VisLineFilter5/5(CentLineValid)
  MATLAB Function4/5(CentLineC0) -> VisLineFilter5/9(CentLineC0)
  MATLAB Function4/9(LeftLineC3) -> VisLineFilter5/13(LeftLineC3)
  MATLAB Function4/6(CentLineRange) -> VisLineFilter5/10(CentLineRange)
  MATLAB Function4/10(LeftLineC2) -> VisLineFilter5/14(LeftLineC2)
  MATLAB Function4/11(LeftLineC1) -> VisLineFilter5/15(LeftLineC1)
  MATLAB Function4/15(LeftLaneAvail) -> VisLineFilter5/19(LeftLaneAvail)
  MATLAB Function4/12(LeftLineC0) -> VisLineFilter5/16(LeftLineC0)
  MATLAB Function4/16(RightLineValid) -> VisLineFilter5/20(RightLineValid)
  MATLAB Function4/13(LeftLineRange) -> VisLineFilter5/17(LeftLineRange)
  MATLAB Function4/17(RightLineC3) -> VisLineFilter5/21(RightLineC3)
  MATLAB Function4/18(RightLineC2) -> VisLineFilter5/22(RightLineC2)
  MATLAB Function4/19(RightLineC1) -> VisLineFilter5/23(RightLineC1)
  MATLAB Function4/23(RightLaneAvail) -> VisLineFilter5/27(RightLaneAvail)
  MATLAB Function4/20(RightLineC0) -> VisLineFilter5/24(RightLineC0)
  MATLAB Function4/21(RightLineRange) -> VisLineFilter5/25(RightLineRange)
  MATLAB Function4/14(LeftLineReliable) -> VisLineFilter5/18(LeftLineReliable)
  MATLAB Function4/7(CentLineReliable) -> VisLineFilter5/11(CentLineReliable)
  MATLAB Function4/22(RightLineReliable) -> VisLineFilter5/26(RightLineReliable)
  MATLAB Function4/24(Line_State) -> [Line_State]  "LSM_Line_State"
  VisLineFilter5/1(PathValid) -> Bus Creator12/1
  VisLineFilter5/2(PathA3) -> Bus Creator12/2
  VisLineFilter5/3(PathA2) -> Bus Creator12/3
  VisLineFilter5/4(PathA1) -> Bus Creator12/4
  VisLineFilter5/5(PathA0) -> Bus Creator12/5
  VisLineFilter5/6(PathRange) -> Bus Creator12/6
  VisLineFilter5/7(PathReliable) -> Bus Creator12/7
  VisLineFilter5/8(PathLaneAvail) -> Bus Creator12/8, [PathLaneAvail]  "LSM_PathLaneAvail"
  Bus Creator12/1 -> [CentLine]
  [CentLine] -> Bus Selector6/1
  Selector13/1 -> LineSelect/1(CentLaneValid)
  Selector14/1 -> LineSelect/2(CentLineA3)
  Selector15/1 -> LineSelect/3(CentLineA2)
  Selector16/1 -> LineSelect/4(CentLineA1)
  Selector17/1 -> LineSelect/5(CentLineA0)
  Selector18/1 -> LineSelect/6(CentRange)
  [RoadWidth] -> MATLAB Function4/11(RoadWidth)
  [kap] -> Subsystem5/1(kap)
  vRef4/1 -> Subsystem5/2(vRef)  "LSM_VRef"
  [kap] -> MATLAB Function2/3(kap)
  MATLAB Function2/3(Wij_state) -> Terminator2/1
  [RoadWidth] -> MATLAB Function3/8(RoadWidth)
  vRef9/1 -> VisLineFilter3/2(vRef)  "LSM_VRef"
  [RoadWidth] -> VisLineFilter3/10(RoadWidth)  "LSM_RoadWidth1"
  [kap] -> Subsystem4/1(kap)
  vRef10/1 -> Subsystem4/2(vRef)  "LSM_VRef"
  Unit Delay11/1 -> MATLAB Function6/5(HWAStsK1)
  [HWASts] -> Unit Delay11/1, MATLAB Function6/4(HWASts)
  [kap] -> MATLAB Function5/3(kap)
  MATLAB Function5/3(Wij_state) -> [Wij_State]  "LSM_Wij_State"
  [preDis] -> MATLAB Function4/12(preDis)
  [PathLaneAvail] -> Signal Copy3/1
  [HWASts] -> Subsystem4/21(HWASts)
  [HWASts] -> Subsystem5/21(HWASts)
  LeftLine_Change/1 -> Terminator3/1
  VisLineFilter3/3(RightOffset_b) -> DetectIncrease1/1(RightOffset_b)  "LSM_RightOffset_b"
  DetectIncrease/1(Out) -> [LeftOffset_b]
  DetectIncrease1/1(Out) -> [RightOffset_b]
  RightLine_Change/1 -> Terminator49/1
  VisLineFilter3/2(LeftOffset_b) -> DetectIncrease/1(LeftOffset_b)  "LSM_LeftOffset_b"
  [LH1Wij] -> MATLAB Function3/9(LH1Wij)
  [LH2Wij] -> MATLAB Function3/10(LH2Wij)
  Signal Copy/1 -> Unit Delay16/1, HWALineCalc/3(HWASts)  "LSM_HWASts"
  [TJA_Line_State] -> Signal Copy1/1
  Signal Copy1/1 -> HWALineCalc/2(TJA_Line_State)  "LSM_TJA_Line_State1"
  Signal Copy2/1 -> Unit Delay27/1
  [HWALineC0] -> Signal Copy2/1
  Signal Copy3/1 -> HWALineCalc/11(PathLaneAvail)  "LSM_PathLaneAvail1"
  [TJA_Line] -> Bus Selector2/1
  Bus Selector2/1 -> HWALineCalc/12(TJALineValid)  "<HWALineValid>"
  Bus Selector2/2 -> HWALineCalc/13(TJALineA3)  "<HWALineC3>"
  Bus Selector2/3 -> HWALineCalc/14(TJALineA2)  "<HWALineC2>"
  Bus Selector2/4 -> HWALineCalc/15(TJALineA1)  "<HWALineC1>"
  Bus Selector2/5 -> HWALineCalc/16(TJALineA0)  "<HWALineC0>"
  Bus Selector2/6 -> HWALineCalc/17(TJALineRange)  "<HWARange>"
  Mux14/1 -> [VisEdgeConf]
  Mux10/1 -> [VisEdgeA3]
  Mux11/1 -> [VisEdgeA2]
  Mux12/1 -> [VisEdgeA1]
  Mux13/1 -> [VisEdgeA0]
  Mux9/1 -> [VisEdgeRange]
  Mux15/1 -> [VisEdgeReliable]
  L1_Conf/1 -> Mux/1
  L2_Conf/1 -> Mux/2
  L3_Conf/1 -> Mux/3
  L4_Conf/1 -> Mux/4
  L1_A3/1 -> Mux1/1
  L2_A3/1 -> Mux1/2
  L3_A3/1 -> Mux1/3
  L4_A3/1 -> Mux1/4
  L1_A2/1 -> Mux2/1
  L2_A2/1 -> Mux2/2
  L3_A2/1 -> Mux2/3
  L4_A2/1 -> Mux2/4
  L1_A1/1 -> Mux3/1
  L2_A1/1 -> Mux3/2
  L3_A1/1 -> Mux3/3
  L4_A1/1 -> Mux3/4
  L1_A0/1 -> Mux4/1
  L2_A0/1 -> Mux4/2
  L3_A0/1 -> Mux4/3
  L4_A0/1 -> Mux4/4
  L1_R/1 -> Mux5/1
  L2_R/1 -> Mux5/2
  L3_R/1 -> Mux5/3
  L4_R/1 -> Mux5/4
  L1_Re/1 -> Mux6/1
  L2_Re/1 -> Mux6/2
  L3_Re/1 -> Mux6/3
  L4_Re/1 -> Mux6/4
  LeftLineType1/1 -> Mux7/1
  RightLineType1/1 -> Mux7/2
  LH1Color/1 -> Mux8/1
  LH2Color/1 -> Mux8/2
  Edge1_R/1 -> Mux9/1
  Edge2_R/1 -> Mux9/2
  Edge1_A3/1 -> Mux10/1
  Edge2_A3/1 -> Mux10/2
  Edge1_A2/1 -> Mux11/1
  Edge2_A2/1 -> Mux11/2
  Edge1_A1/1 -> Mux12/1
  Edge2_A1/1 -> Mux12/2
  Edge1_A0/1 -> Mux13/1
  Edge2_A0/1 -> Mux13/2
  Edge1_Conf/1 -> Mux14/1
  Edge2_Conf/1 -> Mux14/2
  Edge1_Re/1 -> Mux15/1
  Edge2_Re/1 -> Mux15/2
